simulink model "untitled1"  (Simulink 7.1)
settings: Solver=ode45  StartTime=0.0  StopTime=50  RelTol=1e-3
libraries: simulink_extras x1
settings Model: Creator=Slavi  LastModifiedBy=Slavi

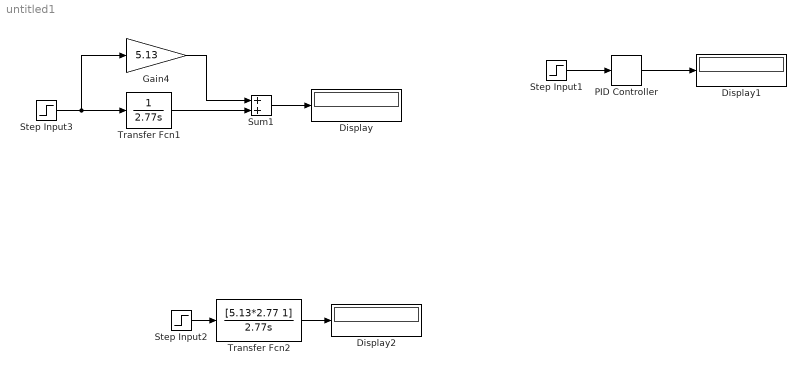
== system untitled1 ==
  Display : Display
  Display1 : Display
  Display2 : Display
  Gain4 : Gain  Gain=5.13  SaturateOnIntegerOverflow=on  OutDataTypeStr=Inherit: Same as input  ParamDataTypeStr=Inherit: Same as input
  PID Controller : simulink_extras/Additional Linear/PID Controller  SystemSampleTime=-1  P=5.13  I=1/2.77  D=0
  Step Input1 : Step  Time=0  After=233  SampleTime=0
  Step Input2 : Step  Time=0  After=233  SampleTime=0
  Step Input3 : Step  Time=0  After=233  SampleTime=0
  Sum1 : Sum  SaturateOnIntegerOverflow=on  InputSameDT=on  OutDataTypeStr=Inherit: Same as first input
  Transfer Fcn1 : TransferFcn  Denominator=[2.77 0]
  Transfer Fcn2 : TransferFcn  Numerator=[5.13*2.77 1]  Denominator=[2.77 0]
  wires:
  Step Input3/1 -> Transfer Fcn1/1, Gain4/1
  Gain4/1 -> Sum1/1
  Transfer Fcn1/1 -> Sum1/2
  Sum1/1 -> Display/1
  Step Input1/1 -> PID Controller/1
  PID Controller/1 -> Display1/1
  Step Input2/1 -> Transfer Fcn2/1
  Transfer Fcn2/1 -> Display2/1
